simulink model "PTO_Model"  (Simulink 7.4)
settings: Solver=ode45  StartTime=0.0  StopTime=end_sim  MaxStep=1e-3  RelTol=1e-3
values from neighbouring files (symbols this model uses):
  A = 1    [PTO_Model_RUN.m]
  A_bore = pi*Dbore^2/4    (= 0.0182414692475)    [PTO_Model_RUN.m]
  A_rod = pi*(Dbore^2-Drod^2)/4    (= 0.0101341495819)    [PTO_Model_RUN.m]
  Gen_Damp = 2.1    [PTO_Model_RUN.m]
  hyd_mot_eff = 0.93    [PTO_Model_RUN.m]
  hyd_mot_tot = 0.865    [PTO_Model_RUN.m]
  Jtot = Jmot+Jgen    (= 3.961)    [PTO_Model_RUN.m]
  p_atm = 101325    [PTO_Model_RUN.m]
  pump_vol_eff = 0.97    [PTO_Model_RUN.m]
  T = 13    [PTO_Model_RUN.m]
  Vg = 0.00025    [PTO_Model_RUN.m]
undefined symbols (not defined in the file or in its folder): p_hp, p_lp, V_hp, V_lp
settings Model: Creator=Relley Ruehl  LastModifiedBy=Relley Ruehl

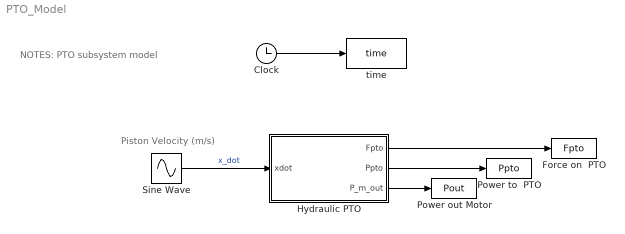
== system PTO_Model ==
  note: Piston Velocity (m/s)
  note: NOTES:
      | PTO subsystem model
  Clock : Clock
      settings: Decimation=10
  Force on  PTO : ToWorkspace  VariableName=Fpto  SampleTime=-1  SaveFormat=Array
  "Hydraulic PTO " : Subsystem
  "Power out Motor " : ToWorkspace  VariableName=Pout  SampleTime=-1  SaveFormat=Array
  Power to  PTO : ToWorkspace  VariableName=Ppto  SampleTime=-1  SaveFormat=Array
  Sine Wave : Sin  Amplitude=A  Bias=0  Frequency=2*pi/T  Phase=pi/2  Samples=10  SampleTime=0  Offset=0
  time : ToWorkspace  VariableName=time  SampleTime=-1  SaveFormat=Array
  wires:
  "Hydraulic PTO "/1(Fpto) -> Force on  PTO/1
  "Hydraulic PTO "/3(P_m_out) -> "Power out Motor "/1
  Clock/1 -> time/1
  Sine Wave/1 -> "Hydraulic PTO "/1(xdot)  "x_dot"
  "Hydraulic PTO "/2(Ppto) -> Power to  PTO/1

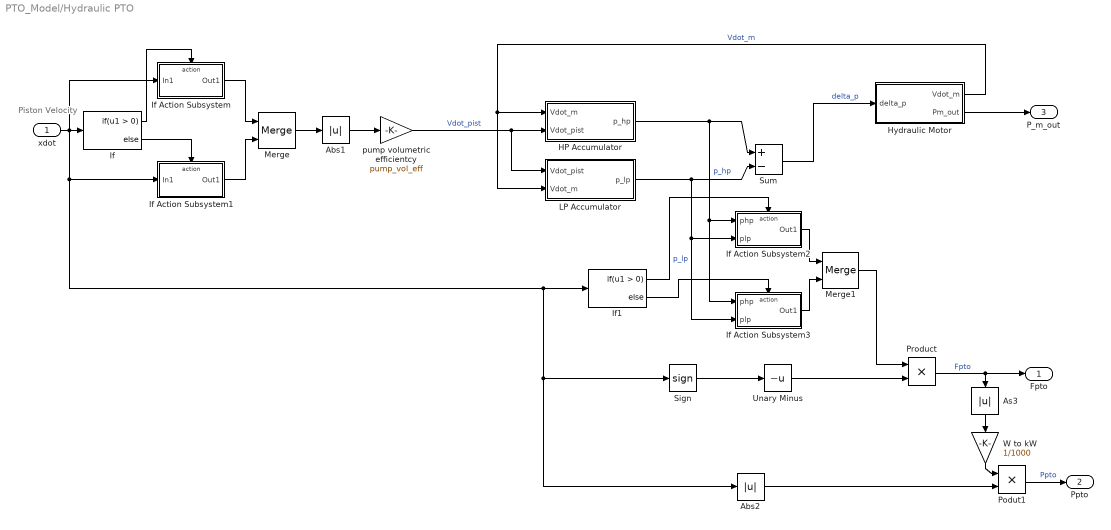
== system PTO_Model/Hydraulic PTO  ==
  note: Piston
      | Velocity
  xdot : Inport
  Abs1 : Abs
  Abs2 : Abs
  As3 : Abs
  HP Accumulator : Subsystem
  Hydraulic Motor : Subsystem
  If : If
  If Action Subsystem : Subsystem  TreatAsAtomicUnit=on
  If Action Subsystem1 : Subsystem  TreatAsAtomicUnit=on
  If Action Subsystem2 : Subsystem  TreatAsAtomicUnit=on
  If Action Subsystem3 : Subsystem  TreatAsAtomicUnit=on
  If1 : If
  LP Accumulator : Subsystem
  Merge : Merge
  Merge1 : Merge
  Podut1 : Product  RndMeth=Zero
  Product : Product  RndMeth=Zero
  Sign : Signum
  Sum : Sum  Inputs=+-
  Unary Minus : UnaryMinus
  W to kW : Gain  Gain=1/1000
  pump volumetric efficientcy : Gain  Gain=pump_vol_eff
  Fpto : Outport
  Ppto : Outport  Port=2
  P_m_out : Outport  Port=3
  wires:
  xdot/1 -> If/1, If Action Subsystem/1(In1), If Action Subsystem1/1(In1), If1/1, Sign/1, Abs2/1
  HP Accumulator/1(p_hp) -> Sum/1, If Action Subsystem2/1(php), If Action Subsystem3/1(php)  "p_hp"
  LP Accumulator/1(p_lp) -> Sum/2, If Action Subsystem2/2(plp), If Action Subsystem3/2(plp)  "p_lp"
  Sum/1 -> Hydraulic Motor/1(delta_p)  "delta_p"
  Hydraulic Motor/2(Pm_out) -> P_m_out/1
  Sign/1 -> Unary Minus/1
  Unary Minus/1 -> Product/2
  Product/1 -> Fpto/1, As3/1  "Fpto"
  Hydraulic Motor/1(Vdot_m) -> LP Accumulator/2(Vdot_m), HP Accumulator/1(Vdot_m)  "Vdot_m"
  If/1 -> If Action Subsystem/Action
  If/2 -> If Action Subsystem1/Action
  pump volumetric efficientcy/1 -> HP Accumulator/2(Vdot_pist), LP Accumulator/1(Vdot_pist)  "Vdot_pist"
  Merge/1 -> Abs1/1
  Abs1/1 -> pump volumetric efficientcy/1
  If1/1 -> If Action Subsystem2/Action
  If1/2 -> If Action Subsystem3/Action
  If Action Subsystem2/1(Out1) -> Merge1/1
  If Action Subsystem3/1(Out1) -> Merge1/2
  If Action Subsystem/1(Out1) -> Merge/1
  If Action Subsystem1/1(Out1) -> Merge/2
  Merge1/1 -> Product/1
  Podut1/1 -> Ppto/1  "Ppto"
  Abs2/1 -> Podut1/2
  As3/1 -> W to kW/1
  W to kW/1 -> Podut1/1

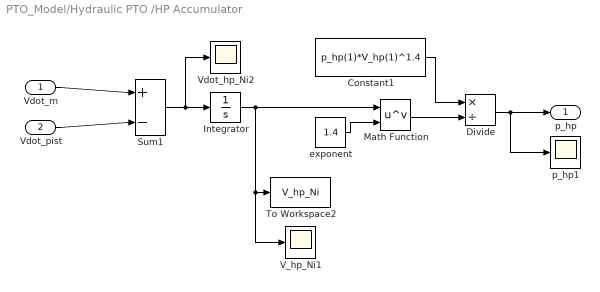
== system PTO_Model/Hydraulic PTO /HP Accumulator ==
  Vdot_m : Inport
  Vdot_pist : Inport  Port=2
  Constant1 : Constant  Value=p_hp(1)*V_hp(1)^1.4
  Divide : Product  Inputs=*/
  Integrator : Integrator  InitialCondition=V_hp(1)
  Math Function : Math  Operator=pow  SaturateOnIntegerOverflow=on
  Sum1 : Sum  Inputs=+|-
  To Workspace2 : ToWorkspace  VariableName=V_hp_Ni  SampleTime=-1  SaveFormat=Array
  V_hp_Ni1 : Scope
      settings: TimeRange=25  YMin=399  YMax=401  SaveName=ScopeData12
  Vdot_hp_Ni2 : Scope
      settings: TimeRange=25  YMin=-1e-015  YMax=1.5e-015  SaveName=ScopeData13
  exponent : Constant  Value=1.4
  p_hp1 : Scope
      settings: TimeRange=50  YMin=16050000  YMax=16110000  SaveName=ScopeData14
  p_hp : Outport
  wires:
  Integrator/1 -> Math Function/1, To Workspace2/1, V_hp_Ni1/1
  Divide/1 -> p_hp1/1, p_hp/1
  Math Function/1 -> Divide/2
  exponent/1 -> Math Function/2
  Constant1/1 -> Divide/1
  Vdot_m/1 -> Sum1/1
  Vdot_pist/1 -> Sum1/2
  Sum1/1 -> Integrator/1, Vdot_hp_Ni2/1

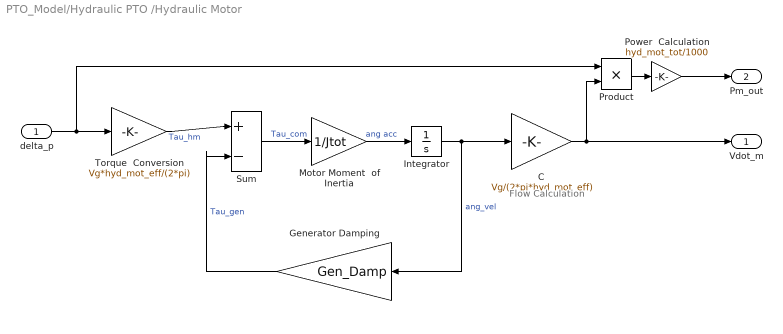
== system PTO_Model/Hydraulic PTO /Hydraulic Motor ==
  note: Flow
      | Calculation
  delta_p : Inport
  C : Gain  Gain=Vg/(2*pi*hyd_mot_eff)
  Generator Damping : Gain  Gain=Gen_Damp
  Integrator : Integrator
  Motor Moment  of Inertia : Gain  Gain=1/Jtot
  Power  Calculation : Gain  Gain=hyd_mot_tot/1000
  Product : Product  RndMeth=Zero
  Sum : Sum  Inputs=|+|-|
  Torque  Conversion : Gain  Gain=Vg*hyd_mot_eff/(2*pi)
  Vdot_m : Outport
  Pm_out : Outport  Port=2
  wires:
  delta_p/1 -> Product/1, Torque  Conversion/1
  Sum/1 -> Motor Moment  of Inertia/1  "Tau_com"
  Motor Moment  of Inertia/1 -> Integrator/1  "ang acc"
  Integrator/1 -> C/1, Generator Damping/1  "ang_vel"
  Torque  Conversion/1 -> Sum/1  "Tau_hm"
  C/1 -> Vdot_m/1, Product/2
  Product/1 -> Power  Calculation/1
  Power  Calculation/1 -> Pm_out/1
  Generator Damping/1 -> Sum/2  "Tau_gen"

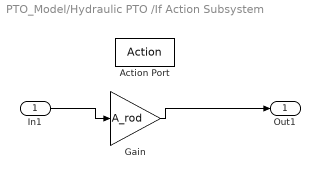
== system PTO_Model/Hydraulic PTO /If Action Subsystem ==
  In1 : Inport
  Action Port : ActionPort  ActionType=then
  Gain : Gain  Gain=A_rod
  Out1 : Outport
  wires:
  In1/1 -> Gain/1
  Gain/1 -> Out1/1

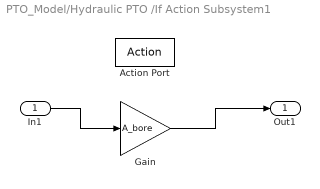
== system PTO_Model/Hydraulic PTO /If Action Subsystem1 ==
  In1 : Inport
  Action Port : ActionPort  ActionType=else
  Gain : Gain  Gain=A_bore
  Out1 : Outport
  wires:
  In1/1 -> Gain/1
  Gain/1 -> Out1/1

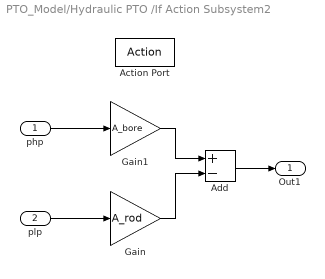
== system PTO_Model/Hydraulic PTO /If Action Subsystem2 ==
  php : Inport
  plp : Inport  Port=2
  Action Port : ActionPort  ActionType=then
  Add : Sum  Inputs=+-
  Gain : Gain  Gain=A_rod
  Gain1 : Gain  Gain=A_bore
  Out1 : Outport
  wires:
  php/1 -> Gain1/1
  plp/1 -> Gain/1
  Gain1/1 -> Add/1
  Gain/1 -> Add/2
  Add/1 -> Out1/1

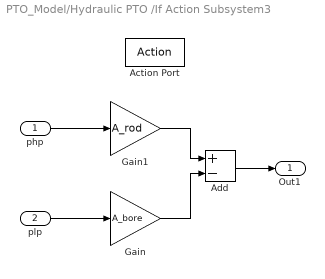
== system PTO_Model/Hydraulic PTO /If Action Subsystem3 ==
  php : Inport
  plp : Inport  Port=2
  Action Port : ActionPort  ActionType=else
  Add : Sum  Inputs=+-
  Gain : Gain  Gain=A_bore
  Gain1 : Gain  Gain=A_rod
  Out1 : Outport
  wires:
  php/1 -> Gain1/1
  plp/1 -> Gain/1
  Gain1/1 -> Add/1
  Gain/1 -> Add/2
  Add/1 -> Out1/1

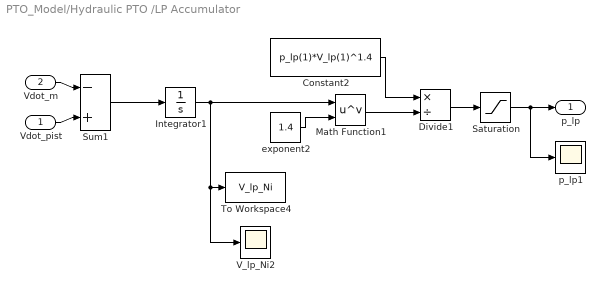
== system PTO_Model/Hydraulic PTO /LP Accumulator ==
  Vdot_pist : Inport
  Vdot_m : Inport  Port=2
  Constant2 : Constant  Value=p_lp(1)*V_lp(1)^1.4
  Divide1 : Product  Inputs=*/
  Integrator1 : Integrator  InitialCondition=V_lp(1)
  Math Function1 : Math  Operator=pow  SaturateOnIntegerOverflow=on
  Saturation : Saturate  UpperLimit=inf  LowerLimit=p_atm
  Sum1 : Sum  Inputs=-|+
  To Workspace4 : ToWorkspace  VariableName=V_lp_Ni  SampleTime=-1  SaveFormat=Array
  V_lp_Ni2 : Scope
      settings: TimeRange=25  YMin=0  YMax=5000
  exponent2 : Constant  Value=1.4
  p_lp1 : Scope
      settings: TimeRange=50  YMin=100000  YMax=110000  SaveName=ScopeData3
  p_lp : Outport
  wires:
  Math Function1/1 -> Divide1/2
  exponent2/1 -> Math Function1/2
  Integrator1/1 -> Math Function1/1, To Workspace4/1, V_lp_Ni2/1
  Constant2/1 -> Divide1/1
  Vdot_m/1 -> Sum1/1
  Vdot_pist/1 -> Sum1/2
  Sum1/1 -> Integrator1/1
  Divide1/1 -> Saturation/1
  Saturation/1 -> p_lp/1, p_lp1/1
